simulink model "Plant_inversion"  (R2017b)
settings: Solver=FixedStepDiscrete  StartTime=0.0  StopTime=10  FixedStep=Ts  RelTol=1e-3
values from neighbouring files (symbols this model uses):
  cd_den_clean = cell2mat(den_clean)    [controller_design.m]
  cd_num_clean = cell2mat(num_clean)    [controller_design.m]
  d_den = cell2mat(sysd.den)    [controller_design.m]
  d_num = cell2mat(sysd.num)    [controller_design.m]
  Ts = 1/fs    (= 0.001)    [demo.m]
settings Model: Creator=hasee  LastModifiedBy=hasee

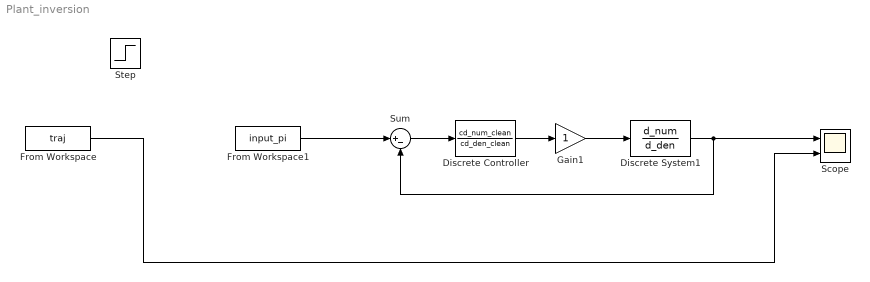
== system Plant_inversion ==
  Discrete Controller : DiscreteTransferFcn  Numerator=cd_num_clean  Denominator=cd_den_clean  SampleTime=Ts
  Discrete System1 : DiscreteTransferFcn  Numerator=d_num  Denominator=d_den
  From Workspace : FromWorkspace  VariableName=traj  SampleTime=0.001
  From Workspace1 : FromWorkspace  VariableName=input_pi  SampleTime=0.001
  Gain1 : Gain
  Scope : Scope  NumInputPorts=2
  Step : Step  After=100  SampleTime=Ts
  Sum : Sum  Inputs=|+-
  wires:
  From Workspace/1 -> Scope/2
  From Workspace1/1 -> Sum/1
  Discrete System1/1 -> Sum/2, Scope/1
  Sum/1 -> Discrete Controller/1
  Discrete Controller/1 -> Gain1/1
  Gain1/1 -> Discrete System1/1
